simulink model "Vasca_NL"  (R2022a)
settings: Solver=VariableStepAuto  StartTime=0.0  StopTime=10.0  RelTol=1e-3
values from neighbouring files (symbols this model uses):
  Area = 0.08    [ControlloVasca.m]
  Au = 43*1e-6    (= 4.3e-05)    [ControlloVasca.m]
  g = 9.8    [ControlloVasca.m]
  hu = -0.095    [ControlloVasca.m]
  L_T = 0:0.01:0.2    [ControlloVasca.m]
  Q_A = 1e-6*[0 8.8 24.6 42.0 57.1 72.4 86.1 102.3 117.6 132.0 144.9]    [ControlloVasca.m]
  Tn_A = 0:0.5:5    [ControlloVasca.m]
  Tn_T = [4.5221 4.4452 4.2412 3.9653 3.7932 3.5179 3.2742 3.0624 2.8349 2.5936 2.3522 2.1423 1.9151 1.6591 1.4251 1.1892 0.9053 0.7329 0.4750 0.2664 0.0471]    [ControlloVasca.m]
  x0 = 0.1    [ControlloVasca.m]
settings Model: LastModifiedBy=cl481357
settings OptimizationCC: BlockReduction=off  BooleanDataType=off
settings DebuggingCC: SaveWithParameterizedLinksMsg=none  UnderspecifiedInitializationDetection=Classic  MergeDetectMultiDrivingBlocksExec=none  SignalResolutionControl=TryResolveAllWithWarning
settings HardwareCC: TargetUnknown=on
settings ModelReferenceCC: PropagateSignalLabelsOutOfModel=off

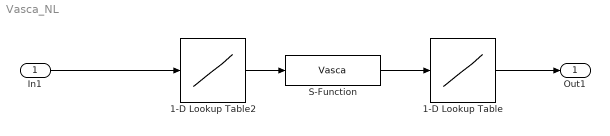
== system Vasca_NL ==
  In1 : Inport
  1-D Lookup Table : Lookup_n-D  NumberOfTableDimensions=1  BreakpointsForDimension1=L_T  Table=Tn_T  InternalRulePriority=Speed  RndMeth=Simplest
  1-D Lookup Table2 : Lookup_n-D  NumberOfTableDimensions=1  BreakpointsForDimension1=Tn_A  Table=Q_A  InternalRulePriority=Speed  RndMeth=Simplest
  S-Function : S-Function  FunctionName=Vasca  Parameters=x0,Area,Au,g,hu  SFunctionDeploymentMode=off  EnableBusSupport=off
  Out1 : Outport
  wires:
  1-D Lookup Table2/1 -> S-Function/1
  S-Function/1 -> 1-D Lookup Table/1
  1-D Lookup Table/1 -> Out1/1
  In1/1 -> 1-D Lookup Table2/1
